simulink library "SINGLE_OPLEV_NOOSEM_MASTER"  (Simulink 8.6)
settings: Solver=ode45  StartTime=0.0  StopTime=10.0  RelTol=1e-3
libraries: cdsEpicsOut x23, cdsFilt x18, VIS_LIB x9, cdsTP x6, cdsFiltCtrl x3, cdsMuxMatrix x3, cdsFunctionCall x3, lockin x2, FOUROSEM_COILOUTF_MASTER x1, rtdemod x1, CRYP_TM_MASTER x1, QPD x1
(part 1 of 2)
settings Model: Creator=controls  LastModifiedBy=controls

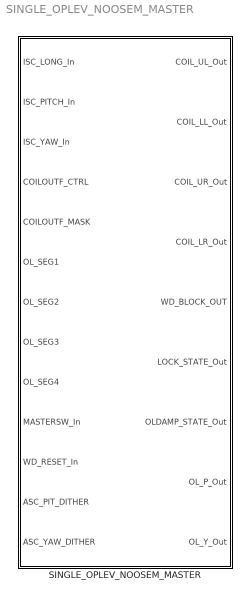
== system SINGLE_OPLEV_NOOSEM_MASTER ==
  SINGLE_OPLEV_NOOSEM_MASTER : Subsystem

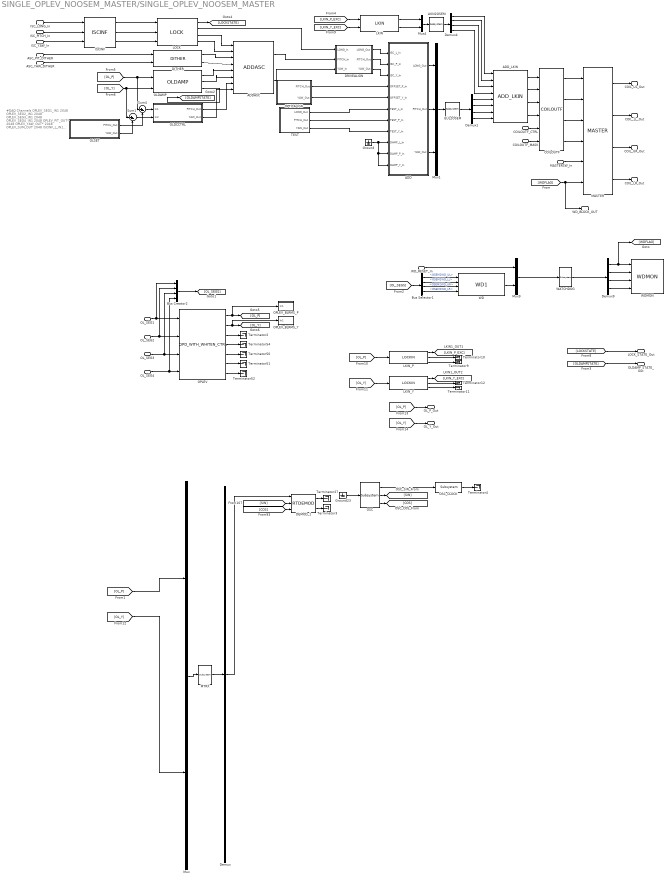
== system SINGLE_OPLEV_NOOSEM_MASTER/SINGLE_OPLEV_NOOSEM_MASTER ==
  note: #DAQ Channels
      | OPLEV_SEG1_IN1 2048
      | OPLEV_SEG2_IN1 2048
      | OPLEV_SEG3_IN1 2048
      | OPLEV_SEG4_IN1 2048
      | OPLEV_PIT_OUT* 2048
      | OPLEV_YAW_OUT* 2048
      | OPLEV_SUM_OUT 2048
      | ISCINF_L_IN1 2048
  ISC_LONG_In : Inport
  ISC_PITCH_In : Inport  Port=2
  ISC_YAW_In : Inport  Port=3
  COILOUTF_CTRL : Inport  Port=4
  COILOUTF_MASK : Inport  Port=5
  OL_SEG1 : Inport  Port=6
  OL_SEG2 : Inport  Port=7
  OL_SEG3 : Inport  Port=8
  OL_SEG4 : Inport  Port=9
  MASTERSW_In : Inport  Port=10
  WD_RESET_In : Inport  Port=11
  ASC_PIT_DITHER : Inport  Port=12
  ASC_YAW_DITHER : Inport  Port=13
  ADD : Subsystem
  ADDASC : VIS_LIB/ADDASC
  ADD_LKIN : VIS_LIB/ADD_LKIN
  Bus Creator2 : BusCreator  Inputs='OSEM2WD_UL','OSEM2WD_LL','OSEM2WD_UR','OSEM2WD_LR'
  Bus Selector1 : BusSelector  OutputSignals=OSEM2WD_UL,OSEM2WD_LL,OSEM2WD_UR,OSEM2WD_LR
  COILOUTF : FOUROSEM_COILOUTF_MASTER/COILOUTF
  DEMOD_1 : rtdemod/RTDEMOD  Tag=top_names
  DITHER : VIS_LIB/DITHER
  DRIVEALIGN : Subsystem
  Demux : Demux  Outputs=1
  Demux1 : Demux
  Demux4 : Demux
  Demux9 : Demux
  EUL2OSEM : cdsMuxMatrix/Subsystem  Tag=cdsMuxMatrix  Description=Any size matrix. Inputs and outputs must be connected using Mux and Demux parts.
      settings: AttributesFormatString=%<Tag>
  Ground : Ground
  Ground23 : Ground
  ISCINF : VIS_LIB/ISCINF
  LKIN : VIS_LIB/LKIN
  LKIN2OSEM : cdsMuxMatrix/Subsystem  Tag=cdsMuxMatrix  Description=Any size matrix. Inputs and outputs must be connected using Mux and Demux parts.
      settings: AttributesFormatString=%<Tag>
  LKIN_P : lockin/LOCKIN  Description=ADL=LOCKIN.adl
      settings: AttributesFormatString=%<Tag>
  LKIN_Y : lockin/LOCKIN  Description=ADL=LOCKIN.adl
      settings: AttributesFormatString=%<Tag>
  LOCK : VIS_LIB/LOCK
  MASTER : CRYP_TM_MASTER/CRYP_TM_MASTER/MASTER
  MTRX : cdsMuxMatrix/Subsystem  Tag=cdsMuxMatrix  Description=Any size matrix. Inputs and outputs must be connected using Mux and Demux parts.
      settings: AttributesFormatString=%<Tag>
  Mux : Mux  Inputs=2
  Mux1 : Mux  Inputs=3
  Mux4 : Mux  Inputs=2
  Mux9 : Mux  Inputs=2
  OLDAMP : VIS_LIB/OLDAMP
  OLDCCTRL : Subsystem
  OLSET : Subsystem  AncestorBlock=SINGLE_OPLEV_NOOSEM_MASTER/SINGLE_OPLEV_NOOSEM_MASTER/OLDCCTRL
  OPLEV : QPD/QPD_WITH_WHITEN_CTRL
  OPLEV_BLRMS_P : Subsystem
  OPLEV_BLRMS_Y : Subsystem
  OPTICALIGN : Subsystem
  OSC : cdsOsc/Subsystem  Tag=cdsOsc  Description=Oscillator
      settings: AttributesFormatString=%<Tag>
  OSC_CLOCK : cdsEpicsOut/Subsystem  Tag=cdsEpicsOutput  Description=|
      | Purpose:                                          
      | Output a FE signal to an EPICS channel.           
      |                                                   
      | Operation:                                        
      | Takes input value and passes it to EPICS record.  
      |                                                   
      | Usage:                                            
      | Name the part with the desired EPICS rrecord name.
      settings: AttributesFormatString=%<Tag>
  Sum1 : Sum  Inputs=|+-
  Sum4 : Sum  Inputs=|+-
  TEST : Subsystem
  Terminator{2..4,9..12,27,50..52,54} (12 alike) : Terminator
  WATCHDOG : cdsFunctionCall/Subsystem  Tag=cdsFunctionCall  Description=inline OSEMWATCHDOG /opt/rtcds/userapps/release/vis/common/src/WATCHDOG.c
      settings: AttributesFormatString=%<Tag>\n%<Description>
  WD : VIS_LIB/WD1
  WDMON : VIS_LIB/WDMON
  COIL_UL_Out : Outport
  COIL_LL_Out : Outport  Port=2
  COIL_UR_Out : Outport  Port=3
  COIL_LR_Out : Outport  Port=4
  WD_BLOCK_OUT : Outport  Port=5
  LOCK_STATE_Out : Outport  Port=6
  OLDAMP_STATE_Out : Outport  Port=7
  OL_P_Out : Outport  Port=8
  OL_Y_Out : Outport  Port=9
  wires:
  OPTICALIGN/2(YAW_Out) -> ADD/5(OFFSET_Y_In)
  OPTICALIGN/1(PITCH_Out) -> ADD/4(OFFSET_P_In)
  LOCK/3 -> ADDASC/1
  TEST/3(YAW_Out) -> ADD/8(TEST_Y_In)
  TEST/2(PITCH_Out) -> ADD/7(TEST_P_In)
  TEST/1(LONG_Out) -> ADD/6(TEST_L_In)
  COILOUTF_CTRL/1 -> COILOUTF/5
  COILOUTF_MASK/1 -> COILOUTF/6
  WD_RESET_In/1 -> Mux9/1
  COILOUTF/4 -> MASTER/4
  COILOUTF/3 -> MASTER/3
  COILOUTF/1 -> MASTER/1
  [WDFLAG] -> WD_BLOCK_OUT/1, MASTER/6
  Mux9/1 -> WATCHDOG/1
  WATCHDOG/1 -> Demux9/1
  Demux9/4 -> WDMON/4
  Demux9/3 -> WDMON/3
  Demux9/2 -> WDMON/2
  Demux9/1 -> WDMON/1, [WDFLAG]
  EUL2OSEM/1 -> Demux1/1
  Mux1/1 -> EUL2OSEM/1
  [OL_SEGS] -> Bus Selector1/1
  Bus Selector1/1 -> WD/1  "<OSEM2WD_UL>"
  Bus Selector1/2 -> WD/2  "<OSEM2WD_LL>"
  Bus Selector1/3 -> WD/3  "<OSEM2WD_UR>"
  Bus Selector1/4 -> WD/4  "<OSEM2WD_LR>"
  OL_SEG1/1 -> Bus Creator2/1, OPLEV/1
  OL_SEG2/1 -> Bus Creator2/2, OPLEV/2
  OL_SEG3/1 -> Bus Creator2/3, OPLEV/3
  OL_SEG4/1 -> Bus Creator2/4, OPLEV/4
  ASC_PIT_DITHER/1 -> DITHER/1
  ASC_YAW_DITHER/1 -> DITHER/2
  [OL_P] -> Sum4/1, OLDAMP/1
  [OL_Y] -> Sum1/1, OLDAMP/2
  LOCK/4 -> ADDASC/2
  DITHER/1 -> ADDASC/3
  DITHER/2 -> ADDASC/4
  OLDAMP/1 -> ADDASC/5
  OLDAMP/2 -> ADDASC/6
  ADD/3(YAW_Out) -> Mux1/3
  ADD/2(PITCH_Out) -> Mux1/2
  ADD/1(LONG_Out) -> Mux1/1
  LOCK/2 -> DRIVEALIGN/1(LONG_In)
  ADDASC/1 -> DRIVEALIGN/2(PITCH_In)
  ADDASC/2 -> DRIVEALIGN/3(YAW_In)
  DRIVEALIGN/1(LONG_Out) -> ADD/1(ISC_L_In)
  DRIVEALIGN/2(PITCH_Out) -> ADD/2(ISC_P_In)
  DRIVEALIGN/3(YAW_Out) -> ADD/3(ISC_Y_In)
  OPLEV/2 -> OPLEV_BLRMS_Y/1(In1), [OL_Y]
  OPLEV/1 -> OPLEV_BLRMS_P/1(In1), [OL_P]
  OPLEV/3 -> Terminator2/1
  OLDAMP/3 -> [OLDAMPSTATE]
  OPLEV/4 -> Terminator54/1
  OPLEV/5 -> Terminator50/1
  OPLEV/6 -> Terminator51/1
  OPLEV/7 -> Terminator52/1
  MASTER/1 -> COIL_UL_Out/1
  MASTER/2 -> COIL_LL_Out/1
  MASTER/3 -> COIL_UR_Out/1
  MASTER/4 -> COIL_LR_Out/1
  Mux4/1 -> LKIN2OSEM/1
  LKIN2OSEM/1 -> Demux4/1
  Demux4/1 -> ADD_LKIN/1
  LKIN/1 -> Mux4/1
  LKIN/2 -> Mux4/2
  Demux4/2 -> ADD_LKIN/2
  Demux4/3 -> ADD_LKIN/3
  Demux4/4 -> ADD_LKIN/4
  Demux1/1 -> ADD_LKIN/5
  Demux1/2 -> ADD_LKIN/6
  Demux1/3 -> ADD_LKIN/7
  Demux1/4 -> ADD_LKIN/8
  ADD_LKIN/1 -> COILOUTF/1
  ADD_LKIN/2 -> COILOUTF/2
  ADD_LKIN/3 -> COILOUTF/3
  ADD_LKIN/4 -> COILOUTF/4
  [LOCKSTATE] -> LOCK_STATE_Out/1
  [OLDAMPSTATE] -> OLDAMP_STATE_Out/1
  LOCK/1 -> [LOCKSTATE]
  [OL_P] -> LKIN_P/1
  LKIN_P/2 -> Terminator10/1
  LKIN_P/3 -> Terminator9/1
  LKIN_P/1 -> [LKIN_P_EXC]
  LKIN_Y/1 -> [LKIN_Y_EXC]
  [OL_Y] -> LKIN_Y/1
  LKIN_Y/2 -> Terminator12/1
  LKIN_Y/3 -> Terminator11/1
  [LKIN_P_EXC] -> LKIN/1
  [LKIN_Y_EXC] -> LKIN/2
  WD/1 -> Mux9/2
  ISC_YAW_In/1 -> ISCINF/3
  ISC_LONG_In/1 -> ISCINF/1
  ISC_PITCH_In/1 -> ISCINF/2
  ISCINF/1 -> LOCK/1
  ISCINF/2 -> LOCK/2
  ISCINF/3 -> LOCK/3
  Mux/1 -> MTRX/1
  MTRX/1 -> Demux/1
  Demux/1 -> DEMOD_1/1
  [SIN] -> DEMOD_1/2
  [COS] -> DEMOD_1/3
  DEMOD_1/1 -> Terminator27/1
  DEMOD_1/2 -> Terminator3/1
  Ground23/1 -> OSC/1
  OSC/1 -> OSC_CLOCK/1
  OSC_CLOCK/1 -> Terminator4/1
  OSC/2 -> [SIN]
  OSC/3 -> [COS]
  [OL_P] -> Mux/1
  [OL_Y] -> Mux/2
  [OL_P] -> OL_P_Out/1
  [OL_Y] -> OL_Y_Out/1
  Bus Creator2/1 -> [OL_SEGS]
  Ground/1 -> ADD/10(DAMP_P_In), ADD/11(DAMP_Y_In), ADD/9(DAMP_L_In)
  COILOUTF/2 -> MASTER/2
  MASTERSW_In/1 -> MASTER/5
  OLSET/1(PITCH_Out) -> Sum4/2
  Sum4/1 -> OLDCCTRL/1(In1)
  Sum1/1 -> OLDCCTRL/2(In2)
  OLSET/2(YAW_Out) -> Sum1/2
  OLDCCTRL/1(PITCH_Out) -> ADDASC/7
  OLDCCTRL/2(YAW_Out) -> ADDASC/8

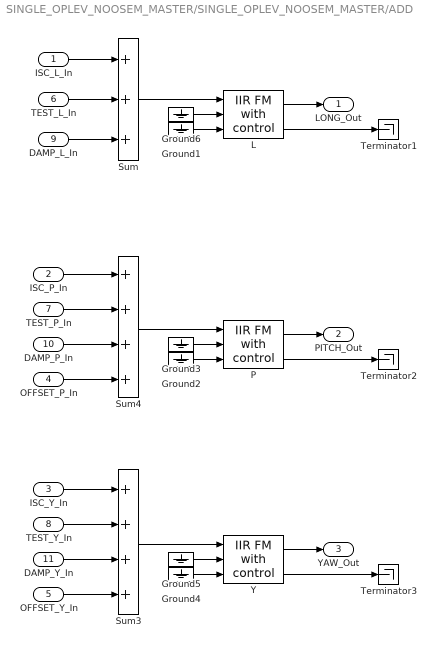
== system SINGLE_OPLEV_NOOSEM_MASTER/SINGLE_OPLEV_NOOSEM_MASTER/ADD ==
  ISC_L_In : Inport
  ISC_P_In : Inport  Port=2
  ISC_Y_In : Inport  Port=3
  OFFSET_P_In : Inport  Port=4
  OFFSET_Y_In : Inport  Port=5
  TEST_L_In : Inport  Port=6
  TEST_P_In : Inport  Port=7
  TEST_Y_In : Inport  Port=8
  DAMP_L_In : Inport  Port=9
  DAMP_P_In : Inport  Port=10
  DAMP_Y_In : Inport  Port=11
  Ground{1..6} (6 alike) : Ground
  L : cdsFiltCtrl/IIR FM with control  Tag=cdsFiltCtrl  Description=|
      | cdsFiltCntrl is the standard IIR filter module (exactly the same as cdsFilt) but with added control data output 'Ctrl'. Filter module digital signal output appears on the first output, which is called 'Val'. 'Ctrl' output has a bit pattern encoding the state of filter's on/off switches (FM1 through FM10). The bit values are:
      |                                                                                                                                                                                                                                                                                                                                       
      | module 	hex	dec                                                                                                                                                                                                                                                                                                                       
      | -----------------------                                                                                                                                                                                                                                                                                                               
      | FM1	0x20                    32                                                                                                                                                                                                                                                                                                        
      | FM2	0x80                     128                                                                                                                                                                                                                                                                                                      
      | FM3	0x200                   512                                                                                                                                                                                                                                                                                                       
      | FM4	0x800                   2048                                                                                                                                                                                                                                                                                                      
      | FM5	0x2000                 8192                                                                                                                                                                                                                                                                                                       
      | FM6	0x8000                 32768                                                                                                                                                                                                                                                                                                      
      | FM7	0x20000                131072                                                                                                                                                                                                                                                                                                     
      | FM8	0x80000                 524288                                                                                                                                                                                                                                                                                                    
      | FM9	0x200000               2097152                                                                                                                                                                                                                                                                                                    
      | FM10	0x800000               8388608                                                                                                                                                                                                                                                                                                   
      |                                                                                                                                                                                                                                                                                                                                       
      | This bit data can be used to drive some other switches or it can be output using a binary I/O module.
      settings: AttributesFormatString=%<Tag>
  P : cdsFiltCtrl/IIR FM with control  Tag=cdsFiltCtrl  Description=|
      | cdsFiltCntrl is the standard IIR filter module (exactly the same as cdsFilt) but with added control data output 'Ctrl'. Filter module digital signal output appears on the first output, which is called 'Val'. 'Ctrl' output has a bit pattern encoding the state of filter's on/off switches (FM1 through FM10). The bit values are:
      |                                                                                                                                                                                                                                                                                                                                       
      | module 	hex	dec                                                                                                                                                                                                                                                                                                                       
      | -----------------------                                                                                                                                                                                                                                                                                                               
      | FM1	0x20                    32                                                                                                                                                                                                                                                                                                        
      | FM2	0x80                     128                                                                                                                                                                                                                                                                                                      
      | FM3	0x200                   512                                                                                                                                                                                                                                                                                                       
      | FM4	0x800                   2048                                                                                                                                                                                                                                                                                                      
      | FM5	0x2000                 8192                                                                                                                                                                                                                                                                                                       
      | FM6	0x8000                 32768                                                                                                                                                                                                                                                                                                      
      | FM7	0x20000                131072                                                                                                                                                                                                                                                                                                     
      | FM8	0x80000                 524288                                                                                                                                                                                                                                                                                                    
      | FM9	0x200000               2097152                                                                                                                                                                                                                                                                                                    
      | FM10	0x800000               8388608                                                                                                                                                                                                                                                                                                   
      |                                                                                                                                                                                                                                                                                                                                       
      | This bit data can be used to drive some other switches or it can be output using a binary I/O module.
      settings: AttributesFormatString=%<Tag>
  Sum : Sum  Inputs=+++
  Sum3 : Sum  Inputs=++++
  Sum4 : Sum  Inputs=++++
  Terminator1 : Terminator
  Terminator2 : Terminator
  Terminator3 : Terminator
  Y : cdsFiltCtrl/IIR FM with control  Tag=cdsFiltCtrl  Description=|
      | cdsFiltCntrl is the standard IIR filter module (exactly the same as cdsFilt) but with added control data output 'Ctrl'. Filter module digital signal output appears on the first output, which is called 'Val'. 'Ctrl' output has a bit pattern encoding the state of filter's on/off switches (FM1 through FM10). The bit values are:
      |                                                                                                                                                                                                                                                                                                                                       
      | module 	hex	dec                                                                                                                                                                                                                                                                                                                       
      | -----------------------                                                                                                                                                                                                                                                                                                               
      | FM1	0x20                    32                                                                                                                                                                                                                                                                                                        
      | FM2	0x80                     128                                                                                                                                                                                                                                                                                                      
      | FM3	0x200                   512                                                                                                                                                                                                                                                                                                       
      | FM4	0x800                   2048                                                                                                                                                                                                                                                                                                      
      | FM5	0x2000                 8192                                                                                                                                                                                                                                                                                                       
      | FM6	0x8000                 32768                                                                                                                                                                                                                                                                                                      
      | FM7	0x20000                131072                                                                                                                                                                                                                                                                                                     
      | FM8	0x80000                 524288                                                                                                                                                                                                                                                                                                    
      | FM9	0x200000               2097152                                                                                                                                                                                                                                                                                                    
      | FM10	0x800000               8388608                                                                                                                                                                                                                                                                                                   
      |                                                                                                                                                                                                                                                                                                                                       
      | This bit data can be used to drive some other switches or it can be output using a binary I/O module.
      settings: AttributesFormatString=%<Tag>
  LONG_Out : Outport
  PITCH_Out : Outport  Port=2
  YAW_Out : Outport  Port=3
  wires:
  OFFSET_P_In/1 -> Sum4/4
  OFFSET_Y_In/1 -> Sum3/4
  DAMP_Y_In/1 -> Sum3/3
  DAMP_P_In/1 -> Sum4/3
  DAMP_L_In/1 -> Sum/3
  ISC_L_In/1 -> Sum/1
  TEST_L_In/1 -> Sum/2
  ISC_Y_In/1 -> Sum3/1
  TEST_Y_In/1 -> Sum3/2
  TEST_P_In/1 -> Sum4/2
  ISC_P_In/1 -> Sum4/1
  Sum/1 -> L/1
  Ground1/1 -> L/3
  Ground6/1 -> L/2
  L/1 -> LONG_Out/1
  Sum4/1 -> P/1
  Ground2/1 -> P/3
  Ground3/1 -> P/2
  P/1 -> PITCH_Out/1
  Sum3/1 -> Y/1
  Ground4/1 -> Y/3
  Ground5/1 -> Y/2
  Y/1 -> YAW_Out/1
  L/2 -> Terminator1/1
  P/2 -> Terminator2/1
  Y/2 -> Terminator3/1

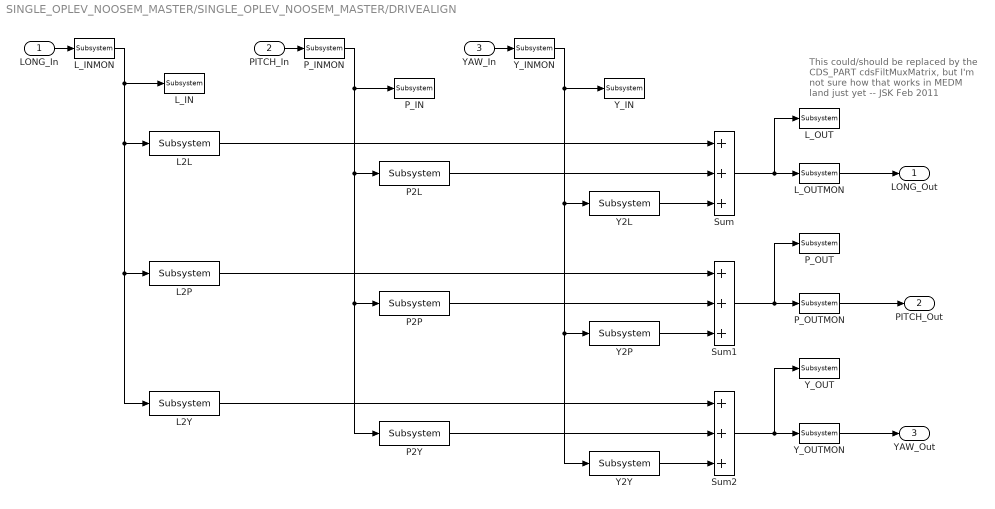
== system SINGLE_OPLEV_NOOSEM_MASTER/SINGLE_OPLEV_NOOSEM_MASTER/DRIVEALIGN ==
  note: This could/should be replaced by
      | the CDS_PART cdsFiltMuxMatrix,
      | but I'm not sure how that works
      | in MEDM land just yet
      | -- JSK Feb 2011
  LONG_In : Inport
  PITCH_In : Inport  Port=2
  YAW_In : Inport  Port=3
  L2L : cdsFilt/Subsystem  Tag=cdsFilt  Description=|
      | Purpose:                                                                                                                                                                                                                                  
      | Standard CDS IIR filter module.                                                                                                                                                                                                           
      |                                                                                                                                                                                                                                           
      | Operation:                                                                                                                                                                                                                                
      | Consists of 10 second order section IIR filters, plus a ramped gain stage. In FE code, also provides pre-defined test points and excitation channel inputs. The filter coefficients are defined in the LIGO system using the 'foton' tool.
      |                                                                                                                                                                                                                                           
      | Usage:                                                                                                                                                                                                                                    
      | Name the part with the desired filter module name.
      settings: AttributesFormatString=%<Tag>
  L2P : cdsFilt/Subsystem  Tag=cdsFilt  Description=|
      | Purpose:                                                                                                                                                                                                                                  
      | Standard CDS IIR filter module.                                                                                                                                                                                                           
      |                                                                                                                                                                                                                                           
      | Operation:                                                                                                                                                                                                                                
      | Consists of 10 second order section IIR filters, plus a ramped gain stage. In FE code, also provides pre-defined test points and excitation channel inputs. The filter coefficients are defined in the LIGO system using the 'foton' tool.
      |                                                                                                                                                                                                                                           
      | Usage:                                                                                                                                                                                                                                    
      | Name the part with the desired filter module name.
      settings: AttributesFormatString=%<Tag>
  L2Y : cdsFilt/Subsystem  Tag=cdsFilt  Description=|
      | Purpose:                                                                                                                                                                                                                                  
      | Standard CDS IIR filter module.                                                                                                                                                                                                           
      |                                                                                                                                                                                                                                           
      | Operation:                                                                                                                                                                                                                                
      | Consists of 10 second order section IIR filters, plus a ramped gain stage. In FE code, also provides pre-defined test points and excitation channel inputs. The filter coefficients are defined in the LIGO system using the 'foton' tool.
      |                                                                                                                                                                                                                                           
      | Usage:                                                                                                                                                                                                                                    
      | Name the part with the desired filter module name.
      settings: AttributesFormatString=%<Tag>
  L_IN : cdsTP/Subsystem  Tag=Test Point
      settings: AttributesFormatString=%<Tag>
  L_INMON : cdsEpicsOut/Subsystem  Tag=cdsEpicsOutput  Description=|
      | Purpose:                                          
      | Output a FE signal to an EPICS channel.           
      |                                                   
      | Operation:                                        
      | Takes input value and passes it to EPICS record.  
      |                                                   
      | Usage:                                            
      | Name the part with the desired EPICS rrecord name.
      settings: AttributesFormatString=%<Tag>
  L_OUT : cdsTP/Subsystem  Tag=Test Point
      settings: AttributesFormatString=%<Tag>
  L_OUTMON : cdsEpicsOut/Subsystem  Tag=cdsEpicsOutput  Description=|
      | Purpose:                                          
      | Output a FE signal to an EPICS channel.           
      |                                                   
      | Operation:                                        
      | Takes input value and passes it to EPICS record.  
      |                                                   
      | Usage:                                            
      | Name the part with the desired EPICS rrecord name.
      settings: AttributesFormatString=%<Tag>
  P2L : cdsFilt/Subsystem  Tag=cdsFilt  Description=|
      | Purpose:                                                                                                                                                                                                                                  
      | Standard CDS IIR filter module.                                                                                                                                                                                                           
      |                                                                                                                                                                                                                                           
      | Operation:                                                                                                                                                                                                                                
      | Consists of 10 second order section IIR filters, plus a ramped gain stage. In FE code, also provides pre-defined test points and excitation channel inputs. The filter coefficients are defined in the LIGO system using the 'foton' tool.
      |                                                                                                                                                                                                                                           
      | Usage:                                                                                                                                                                                                                                    
      | Name the part with the desired filter module name.
      settings: AttributesFormatString=%<Tag>
  P2P : cdsFilt/Subsystem  Tag=cdsFilt  Description=|
      | Purpose:                                                                                                                                                                                                                                  
      | Standard CDS IIR filter module.                                                                                                                                                                                                           
      |                                                                                                                                                                                                                                           
      | Operation:                                                                                                                                                                                                                                
      | Consists of 10 second order section IIR filters, plus a ramped gain stage. In FE code, also provides pre-defined test points and excitation channel inputs. The filter coefficients are defined in the LIGO system using the 'foton' tool.
      |                                                                                                                                                                                                                                           
      | Usage:                                                                                                                                                                                                                                    
      | Name the part with the desired filter module name.
      settings: AttributesFormatString=%<Tag>
  P2Y : cdsFilt/Subsystem  Tag=cdsFilt  Description=|
      | Purpose:                                                                                                                                                                                                                                  
      | Standard CDS IIR filter module.                                                                                                                                                                                                           
      |                                                                                                                                                                                                                                           
      | Operation:                                                                                                                                                                                                                                
      | Consists of 10 second order section IIR filters, plus a ramped gain stage. In FE code, also provides pre-defined test points and excitation channel inputs. The filter coefficients are defined in the LIGO system using the 'foton' tool.
      |                                                                                                                                                                                                                                           
      | Usage:                                                                                                                                                                                                                                    
      | Name the part with the desired filter module name.
      settings: AttributesFormatString=%<Tag>
  P_IN : cdsTP/Subsystem  Tag=Test Point
      settings: AttributesFormatString=%<Tag>
  P_INMON : cdsEpicsOut/Subsystem  Tag=cdsEpicsOutput  Description=|
      | Purpose:                                          
      | Output a FE signal to an EPICS channel.           
      |                                                   
      | Operation:                                        
      | Takes input value and passes it to EPICS record.  
      |                                                   
      | Usage:                                            
      | Name the part with the desired EPICS rrecord name.
      settings: AttributesFormatString=%<Tag>
  P_OUT : cdsTP/Subsystem  Tag=Test Point
      settings: AttributesFormatString=%<Tag>
  P_OUTMON : cdsEpicsOut/Subsystem  Tag=cdsEpicsOutput  Description=|
      | Purpose:                                          
      | Output a FE signal to an EPICS channel.           
      |                                                   
      | Operation:                                        
      | Takes input value and passes it to EPICS record.  
      |                                                   
      | Usage:                                            
      | Name the part with the desired EPICS rrecord name.
      settings: AttributesFormatString=%<Tag>
  Sum : Sum  Inputs=+++
  Sum1 : Sum  Inputs=+++
  Sum2 : Sum  Inputs=+++
  Y2L : cdsFilt/Subsystem  Tag=cdsFilt  Description=|
      | Purpose:                                                                                                                                                                                                                                  
      | Standard CDS IIR filter module.                                                                                                                                                                                                           
      |                                                                                                                                                                                                                                           
      | Operation:                                                                                                                                                                                                                                
      | Consists of 10 second order section IIR filters, plus a ramped gain stage. In FE code, also provides pre-defined test points and excitation channel inputs. The filter coefficients are defined in the LIGO system using the 'foton' tool.
      |                                                                                                                                                                                                                                           
      | Usage:                                                                                                                                                                                                                                    
      | Name the part with the desired filter module name.
      settings: AttributesFormatString=%<Tag>
  Y2P : cdsFilt/Subsystem  Tag=cdsFilt  Description=|
      | Purpose:                                                                                                                                                                                                                                  
      | Standard CDS IIR filter module.                                                                                                                                                                                                           
      |                                                                                                                                                                                                                                           
      | Operation:                                                                                                                                                                                                                                
      | Consists of 10 second order section IIR filters, plus a ramped gain stage. In FE code, also provides pre-defined test points and excitation channel inputs. The filter coefficients are defined in the LIGO system using the 'foton' tool.
      |                                                                                                                                                                                                                                           
      | Usage:                                                                                                                                                                                                                                    
      | Name the part with the desired filter module name.
      settings: AttributesFormatString=%<Tag>
  Y2Y : cdsFilt/Subsystem  Tag=cdsFilt  Description=|
      | Purpose:                                                                                                                                                                                                                                  
      | Standard CDS IIR filter module.                                                                                                                                                                                                           
      |                                                                                                                                                                                                                                           
      | Operation:                                                                                                                                                                                                                                
      | Consists of 10 second order section IIR filters, plus a ramped gain stage. In FE code, also provides pre-defined test points and excitation channel inputs. The filter coefficients are defined in the LIGO system using the 'foton' tool.
      |                                                                                                                                                                                                                                           
      | Usage:                                                                                                                                                                                                                                    
      | Name the part with the desired filter module name.
      settings: AttributesFormatString=%<Tag>
  Y_IN : cdsTP/Subsystem  Tag=Test Point
      settings: AttributesFormatString=%<Tag>
  Y_INMON : cdsEpicsOut/Subsystem  Tag=cdsEpicsOutput  Description=|
      | Purpose:                                          
      | Output a FE signal to an EPICS channel.           
      |                                                   
      | Operation:                                        
      | Takes input value and passes it to EPICS record.  
      |                                                   
      | Usage:                                            
      | Name the part with the desired EPICS rrecord name.
      settings: AttributesFormatString=%<Tag>
  Y_OUT : cdsTP/Subsystem  Tag=Test Point
      settings: AttributesFormatString=%<Tag>
  Y_OUTMON : cdsEpicsOut/Subsystem  Tag=cdsEpicsOutput  Description=|
      | Purpose:                                          
      | Output a FE signal to an EPICS channel.           
      |                                                   
      | Operation:                                        
      | Takes input value and passes it to EPICS record.  
      |                                                   
      | Usage:                                            
      | Name the part with the desired EPICS rrecord name.
      settings: AttributesFormatString=%<Tag>
  LONG_Out : Outport
  PITCH_Out : Outport  Port=2
  YAW_Out : Outport  Port=3
  wires:
  Y_OUTMON/1 -> YAW_Out/1
  P_OUTMON/1 -> PITCH_Out/1
  L_OUTMON/1 -> LONG_Out/1
  Y_INMON/1 -> Y_IN/1, Y2L/1, Y2Y/1, Y2P/1
  P_INMON/1 -> P_IN/1, P2L/1, P2Y/1, P2P/1
  L_INMON/1 -> L_IN/1, L2Y/1, L2P/1, L2L/1
  L2L/1 -> Sum/1
  P2L/1 -> Sum/2
  Y2L/1 -> Sum/3
  Y2P/1 -> Sum1/3
  P2P/1 -> Sum1/2
  L2P/1 -> Sum1/1
  Y2Y/1 -> Sum2/3
  P2Y/1 -> Sum2/2
  L2Y/1 -> Sum2/1
  Sum/1 -> L_OUT/1, L_OUTMON/1
  Sum1/1 -> P_OUT/1, P_OUTMON/1
  Sum2/1 -> Y_OUT/1, Y_OUTMON/1
  LONG_In/1 -> L_INMON/1
  PITCH_In/1 -> P_INMON/1
  YAW_In/1 -> Y_INMON/1
